simulink model "task6"  (R2020a)
settings: Solver=VariableStepAuto  StartTime=0.0  StopTime=5.0  RelTol=1e-3
values from neighbouring files (symbols this model uses):
  Kd = 50    [task6_script.m]
  Kp = 100    [task6_script.m]
undefined symbols (not defined in the file or in its folder): transl, troty
libraries: roblocks x8
settings Model: Creator=root  LastModifiedBy=root

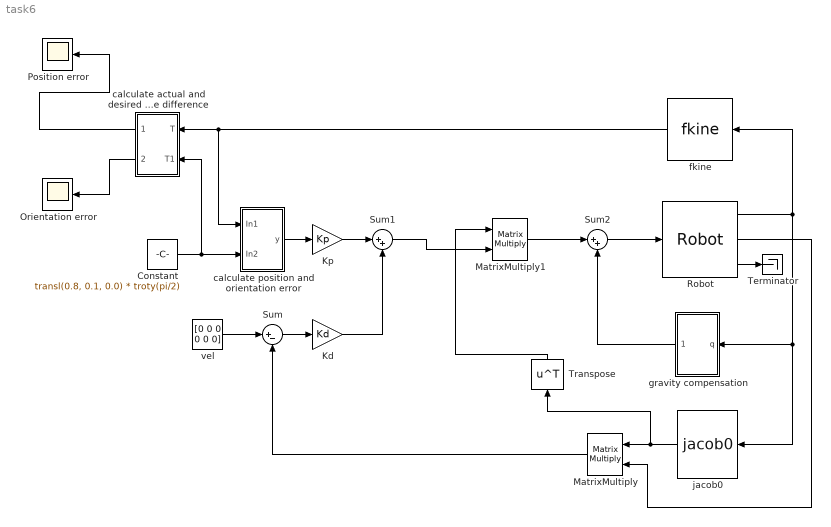
== system task6 ==
  Constant : Constant  Value=transl(0.8, 0.1, 0.0) * troty(pi/2)
  Kd : Gain  Gain=Kd
  Kp : Gain  Gain=Kp
  MatrixMultiply : Product  Multiplication=Matrix(*)
  MatrixMultiply1 : Product  Multiplication=Matrix(*)
  Orientation error : Scope
  Position error : Scope
  Robot : roblocks/Arm/Robot  robot=p560.nofriction  q0=[0 0 0 0 0 0]
  Sum : Sum  Inputs=|+-
  Sum1 : Sum  Inputs=|++
  Sum2 : Sum  Inputs=|++
  Terminator : Terminator
  Transpose : Math  Operator=transpose  SaturateOnIntegerOverflow=on
  calculate actual and desired pose difference : Subsystem
  calculate position and orientation error : Subsystem
  fkine : roblocks/Arm/fkine  robot=p560.nofriction
  gravity compensation : Subsystem
  "jacob0 " : roblocks/Arm/jacob0   robot=p560.nofriction
  vel : Constant  Value=[0 0 0 0 0 0]
  wires:
  vel/1 -> Sum/1
  Sum/1 -> Kd/1
  Constant/1 -> calculate actual and desired pose difference/2(T1), calculate position and orientation error/2(In2)
  calculate position and orientation error/1(y) -> Kp/1
  Kp/1 -> Sum1/1
  Kd/1 -> Sum1/2
  Robot/1 -> fkine/1, "jacob0 "/1, gravity compensation/1(q)
  "jacob0 "/1 -> Transpose/1, MatrixMultiply/1
  Robot/2 -> MatrixMultiply/2
  MatrixMultiply/1 -> Sum/2
  Robot/3 -> Terminator/1
  fkine/1 -> calculate actual and desired pose difference/1(T), calculate position and orientation error/1(In1)
  Transpose/1 -> MatrixMultiply1/1
  Sum1/1 -> MatrixMultiply1/2
  Sum2/1 -> Robot/1
  MatrixMultiply1/1 -> Sum2/1
  gravity compensation/1(Out1) -> Sum2/2
  calculate actual and desired pose difference/1(Out1) -> Position error/1
  calculate actual and desired pose difference/2(Out2) -> Orientation error/1

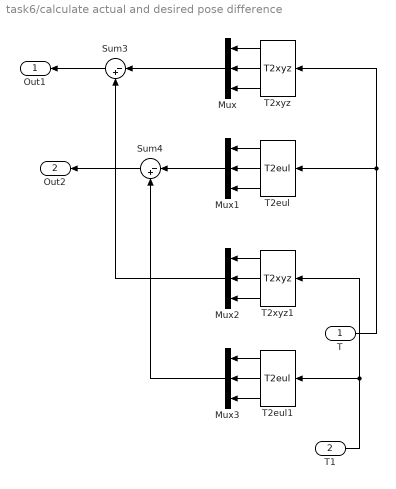
== system task6/calculate actual and desired pose difference ==
  T : Inport
  T1 : Inport  Port=2
  Mux{,1..3} (4 alike) : Mux  Inputs=3
  Sum3 : Sum  Inputs=|-+
  Sum4 : Sum  Inputs=|-+
  T2eul : roblocks/Toolbox/T2eul  degrees=off
  T2eul1 : roblocks/Toolbox/T2eul  degrees=off
  T2xyz : roblocks/Toolbox/T2xyz
  T2xyz1 : roblocks/Toolbox/T2xyz
  Out1 : Outport
  Out2 : Outport  Port=2
  wires:
  T2xyz1/2 -> Mux2/2
  T2eul1/2 -> Mux3/2
  Sum3/1 -> Out1/1
  Mux3/1 -> Sum4/2
  Mux2/1 -> Sum3/2
  T2xyz/1 -> Mux/1
  T2xyz/2 -> Mux/2
  T2eul/2 -> Mux1/2
  T/1 -> T2eul/1, T2xyz/1
  T2eul/3 -> Mux1/3
  T2xyz1/1 -> Mux2/1
  T2xyz/3 -> Mux/3
  T2xyz1/3 -> Mux2/3
  T2eul1/3 -> Mux3/3
  Mux/1 -> Sum3/1
  T1/1 -> T2eul1/1, T2xyz1/1
  Mux1/1 -> Sum4/1
  Sum4/1 -> Out2/1
  T2eul/1 -> Mux1/1
  T2eul1/1 -> Mux3/1

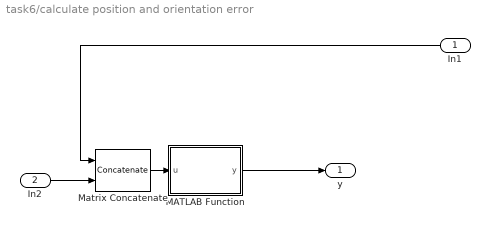
== system task6/calculate position and orientation error ==
  In1 : Inport
  In2 : Inport  Port=2
  MATLAB Function : MATLAB Function  TreatAsAtomicUnit=on
  Matrix Concatenate : Concatenate  Mode=Multidimensional array  ConcatenateDimension=2
  y : Outport
  wires:
  In2/1 -> Matrix Concatenate/2
  Matrix Concatenate/1 -> MATLAB Function/1(u)
  In1/1 -> Matrix Concatenate/1
  MATLAB Function/1(y) -> y/1

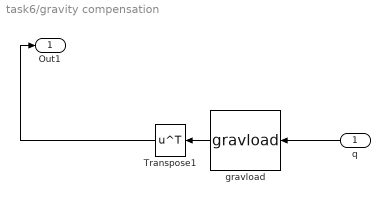
== system task6/gravity compensation ==
  q : Inport
  Transpose1 : Math  Operator=transpose  SaturateOnIntegerOverflow=on
  gravload : roblocks/Arm/gravload  robot=p560.nofriction
  Out1 : Outport
  wires:
  q/1 -> gravload/1
  gravload/1 -> Transpose1/1
  Transpose1/1 -> Out1/1

== matlab function task6/calculate position and orientation error/MATLAB Function ==
  data: u input; y output
function y = fcn(u)

T  = u(1:4, 1:4); % get feedback transformation matrix
Td = u(1:4, 5:8); % get desired transformation matrix

% extract translation parts
p  = T(1:3, 4);
pd = Td(1:3, 4);

% extract rotation parts
n = T(1:3, 1);
o = T(1:3, 2);
a = T(1:3, 3);

nd = Td(1:3, 1);
od = Td(1:3, 2);
ad = Td(1:3, 3);

% Calculate linear position error
ep = pd - p;

% Calculate orientation error
eo = (cross(n, nd) + cross(o, od) + cross(a, ad)) / 2.0;

ex = [ep; eo];

y = ex;
